simulink model "lab7_t20"  (R2021a)
settings: Solver=VariableStepAuto  StartTime=0.0  StopTime=10.0  RelTol=1e-3
libraries: simulink x1
settings Model: Creator=reemb  LastModifiedBy=reemb

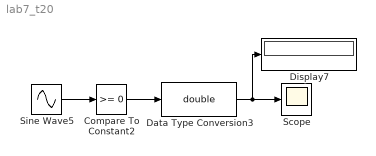
== system lab7_t20 ==
  Compare To Constant2 : simulink/Logic and Bit Operations/Compare To Constant  relop=>=  const=0  OutDataTypeStr=boolean
  Data Type Conversion3 : DataTypeConversion  OutDataTypeStr=double
  Display7 : Display
  Scope : Scope
  Sine Wave5 : Sin  SampleTime=0
  wires:
  Sine Wave5/1 -> Compare To Constant2/1
  Data Type Conversion3/1 -> Display7/1, Scope/1
  Compare To Constant2/1 -> Data Type Conversion3/1
